simulink model "IP_Fuzzy"  (Simulink 5.0)
settings: Solver=ode1  SolverMode=SingleTasking  StartTime=0.0  StopTime=70.0  FixedStep=0.001  RelTol=1e-3
undefined symbols (not defined in the file or in its folder): u1, u2
libraries: pci1711 x3, simulink x2
CloseFcn:
  | rtwprivate ssgencode ModelCloseRequest InvertedPD
settings Model: LastModifiedBy=AD  ExtModeMexFile=rtwinext  ExtModeTrigMode=oneshot  ExtModeTrigDuration=100000  ExtModeLogAll=off  SimulationMode=external  LimitDataPoints=off  BlockReductionOpt=off  BooleanDataType=off  RTWSystemTargetFile=rtwinfbk.tlc  RTWTemplateMakefile=winfbktmf  RTWOptions="-aCCOptimize=1 -aEnforceIntegerDowncast=1 -aExtMode=1 -aFoldNonRolledExpr=1 -aForceParamTrailComments=0 -aGenerateComments=1 -aGenerateReport=0 -aIncDataTypeInIds=0 -aIncHierarchyInIds=0 -aInlineInvariantSignals=0 -aInlineParameters=0 -aInlinedPrmAccess=\"Literals\" -aLocalBlockOutputs=1 -aMaxRTWIdLen=31 -aPrefixModelToSubsysFcnNames=1 -aRTWVerbose=1 -aRebuildAll=0 -aRollThreshold=5 -aShowEliminatedStatements=1"

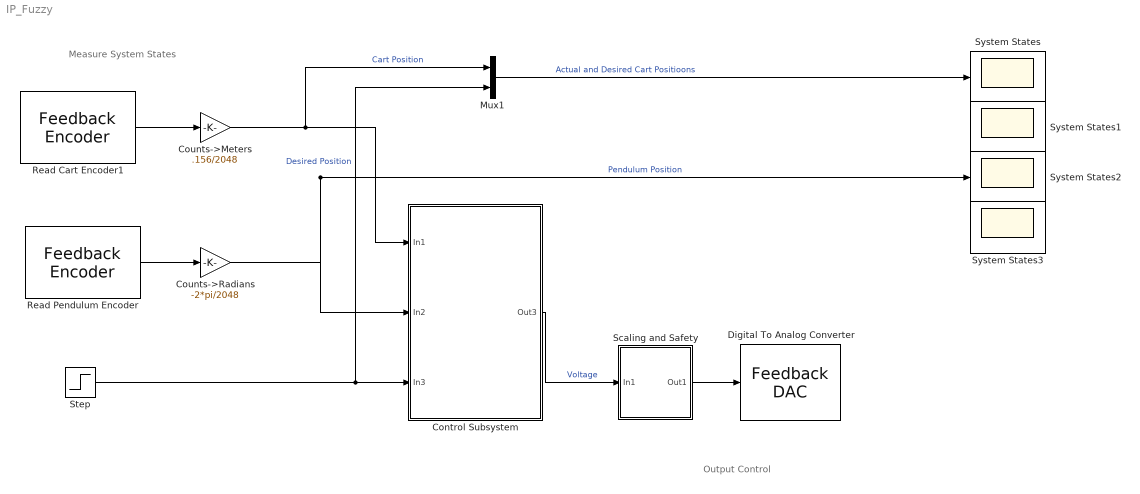
== system IP_Fuzzy ==
  note: Measure System States
  note: Output Control
  Control Subsystem : Subsystem
  Counts->Meters : Gain  Gain=.156/2048  SaturateOnIntegerOverflow=on
  Counts->Radians : Gain  Gain=-2*pi/2048  SaturateOnIntegerOverflow=on
  Digital To Analog Converter : pci1711/Advantech  PCI1711 I//O Board Lib/Feedback DAC  channel=0  range=0  tsamp=0.001  hwAccess=on
  Mux1 : Mux  Inputs=2
  Read Cart Encoder1 : pci1711/Advantech  PCI1711 I//O Board Lib/Feedback Encoder   channel=0  offset=0  tsamp=0.001  hwAccess=on
  Read Pendulum Encoder : pci1711/Advantech  PCI1711 I//O Board Lib/Feedback Encoder   channel=1  offset=-1024  tsamp=0.001  hwAccess=on
  Scaling and Safety : Subsystem
  Step : Step  Time=20  After=0.2  SampleTime=0
  System States{,1..3} (4 alike) : Scope
      System States settings: TimeRange=50  YMin=-0.025  YMax=0.45  SaveName=y  Decimation=0.1  SampleInput=on  SampleTime=0.01
      System States1 settings: TimeRange=50  YMin=-0.125  YMax=0.025  SaveName=y1  Decimation=0.1  SampleInput=on  SampleTime=0.01
      System States2 settings: TimeRange=50  YMin=-0.125  YMax=0.025  SaveName=y2  Decimation=0.1  SampleInput=on  SampleTime=0.01
      System States3 settings: TimeRange=50  YMin=-0.125  YMax=0.025  SaveName=y3  Decimation=0.1  SampleInput=on  SampleTime=0.01
  wires:
  Counts->Meters/1 -> Mux1/1, Control Subsystem/1(In1)  "Cart Position"
  Counts->Radians/1 -> Control Subsystem/2(In2), System States2/1  "Pendulum Position"
  Scaling and Safety/1(Out1) -> Digital To Analog Converter/1
  Step/1 -> Mux1/2, Control Subsystem/3(In3)  "Desired Position"
  Control Subsystem/1(Out3) -> Scaling and Safety/1(In1)  "Voltage"
  Mux1/1 -> System States/1  "Actual and Desired Cart Positioons"
  Read Cart Encoder1/1 -> Counts->Meters/1
  Read Pendulum Encoder/1 -> Counts->Radians/1

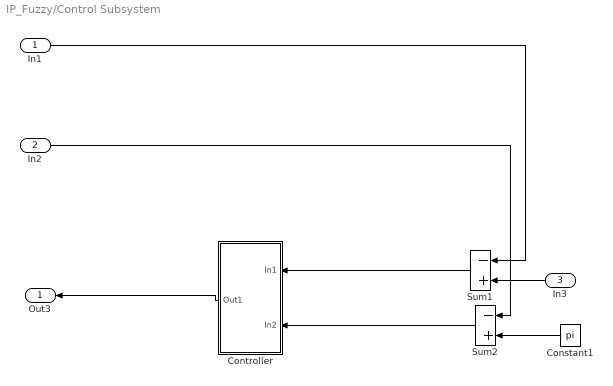
== system IP_Fuzzy/Control Subsystem ==
  In1 : Inport
  In2 : Inport  Port=2
  In3 : Inport  Orientation=left  Port=3
  Constant1 : Constant  Orientation=left  Value=pi
  Controller : Subsystem  Orientation=left
  Sum1 : Sum  Orientation=left  Inputs=-+  SaturateOnIntegerOverflow=on  InputSameDT=on
  Sum2 : Sum  Orientation=left  Inputs=-+  SaturateOnIntegerOverflow=on  InputSameDT=on
  Out3 : Outport  Orientation=left
  wires:
  Controller/1(Out1) -> Out3/1
  Sum1/1 -> Controller/1(In1)
  Sum2/1 -> Controller/2(In2)
  Constant1/1 -> Sum2/2
  In3/1 -> Sum1/2
  In1/1 -> Sum1/1
  In2/1 -> Sum2/1

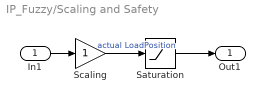
== system IP_Fuzzy/Scaling and Safety ==
  In1 : Inport
  Saturation : Saturate  UpperLimit=2.5  LowerLimit=-2.5
  Scaling : Gain  SaturateOnIntegerOverflow=on
  Out1 : Outport
  wires:
  Saturation/1 -> Out1/1
  In1/1 -> Scaling/1
  Scaling/1 -> Saturation/1  "actual LoadPosition"

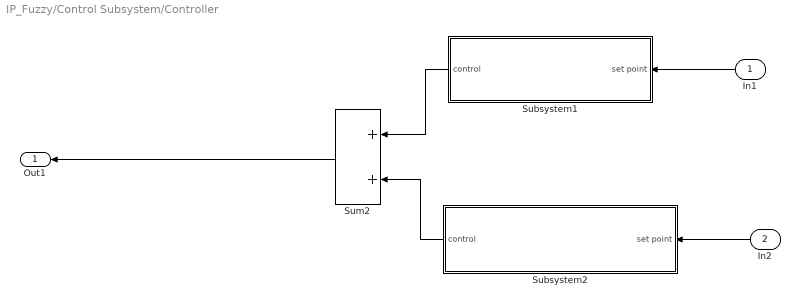
== system IP_Fuzzy/Control Subsystem/Controller ==
  In1 : Inport  Orientation=left
  In2 : Inport  Orientation=left  Port=2
  Subsystem1 : Subsystem  Orientation=left
  Subsystem2 : Subsystem  Orientation=left
  Sum2 : Sum  Orientation=left  SaturateOnIntegerOverflow=on  InputSameDT=on
  Out1 : Outport  Orientation=left
  wires:
  Subsystem1/1(control) -> Sum2/1
  Subsystem2/1(control) -> Sum2/2
  Sum2/1 -> Out1/1
  In1/1 -> Subsystem1/1(set point)
  In2/1 -> Subsystem2/1(set point)

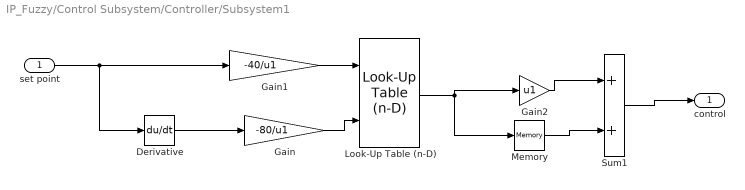
== system IP_Fuzzy/Control Subsystem/Controller/Subsystem1 ==
  set point : Inport
  Derivative : Derivative
  Gain : Gain  Gain=-80/u1  SaturateOnIntegerOverflow=on
  Gain1 : Gain  Gain=-40/u1  SaturateOnIntegerOverflow=on
  Gain2 : Gain  Gain=u1  SaturateOnIntegerOverflow=on
  Look-Up Table (n-D) : simulink/Look-Up Tables/Look-Up Table (n-D)  numDimsPopupSelect=2  bp1=-2:.05:2  bp2=-2:.05:2  bp3=[1:3]  bp4=[1:3]  bpcell={ [1:3], [1:3] }  explicitNumDims=2  searchMode=Binary Search  cacheBpFlag=off  vectorInputFlag=off  tableData=P  interpMethod=Linear  extrapMethod=Linear  rangeErrorMode=None
  Memory : Memory  InheritSampleTime=on
  Sum1 : Sum  SaturateOnIntegerOverflow=on
  control : Outport
  wires:
  Memory/1 -> Sum1/2
  Derivative/1 -> Gain/1
  Gain1/1 -> Look-Up Table (n-D)/1
  Gain/1 -> Look-Up Table (n-D)/2
  Look-Up Table (n-D)/1 -> Gain2/1, Memory/1
  Gain2/1 -> Sum1/1
  Sum1/1 -> control/1
  set point/1 -> Gain1/1, Derivative/1

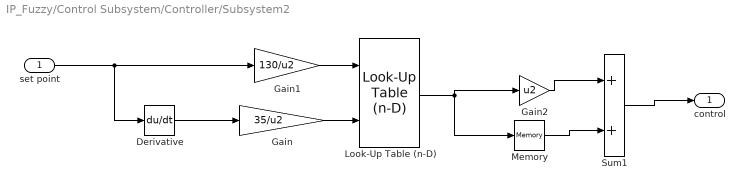
== system IP_Fuzzy/Control Subsystem/Controller/Subsystem2 ==
  set point : Inport
  Derivative : Derivative
  Gain : Gain  Gain=35/u2  SaturateOnIntegerOverflow=on
  Gain1 : Gain  Gain=130/u2  SaturateOnIntegerOverflow=on
  Gain2 : Gain  Gain=u2  SaturateOnIntegerOverflow=on
  Look-Up Table (n-D) : simulink/Look-Up Tables/Look-Up Table (n-D)  numDimsPopupSelect=2  bp1=-2:.05:2  bp2=-2:.05:2  bp3=[1:3]  bp4=[1:3]  bpcell={ [1:3], [1:3] }  explicitNumDims=2  searchMode=Binary Search  cacheBpFlag=off  vectorInputFlag=off  tableData=P  interpMethod=Linear  extrapMethod=Linear  rangeErrorMode=None
  Memory : Memory  InheritSampleTime=on
  Sum1 : Sum  SaturateOnIntegerOverflow=on
  control : Outport
  wires:
  Memory/1 -> Sum1/2
  Derivative/1 -> Gain/1
  Gain1/1 -> Look-Up Table (n-D)/1
  Gain/1 -> Look-Up Table (n-D)/2
  Look-Up Table (n-D)/1 -> Gain2/1, Memory/1
  Gain2/1 -> Sum1/1
  Sum1/1 -> control/1
  set point/1 -> Gain1/1, Derivative/1
